simulink model "SVFB"  (R2024a)
settings: Solver=ode45  StartTime=0.0  StopTime=Tf  RelTol=1e-3
values from neighbouring files (symbols this model uses):
  A = [0 1; 880.87 0]    [main.m]
  B = [0; -9.9453]    [main.m]
  C = [708.27 0]    [main.m]
  K0 = place(A, B, p_desired_tracking)    [main.m]
  L_luemb = place(A', C', desired_poles)'    [main.m]
  S0_x0 = [10 0]'    [main.m]
undefined symbols (not defined in the file or in its folder): err
settings Model: Creator=aless  LastModifiedBy=Stefano

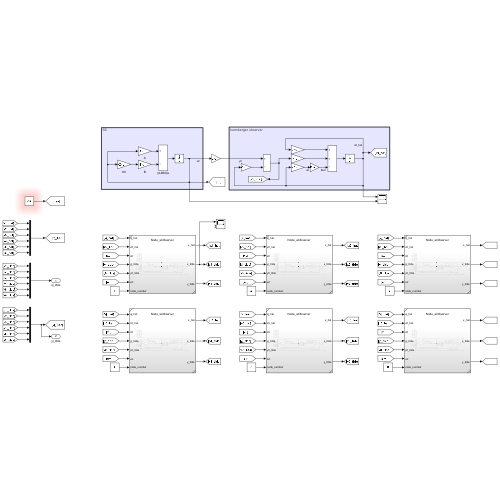
[thumbnail: Simulink's stored preview of the top-level diagram]
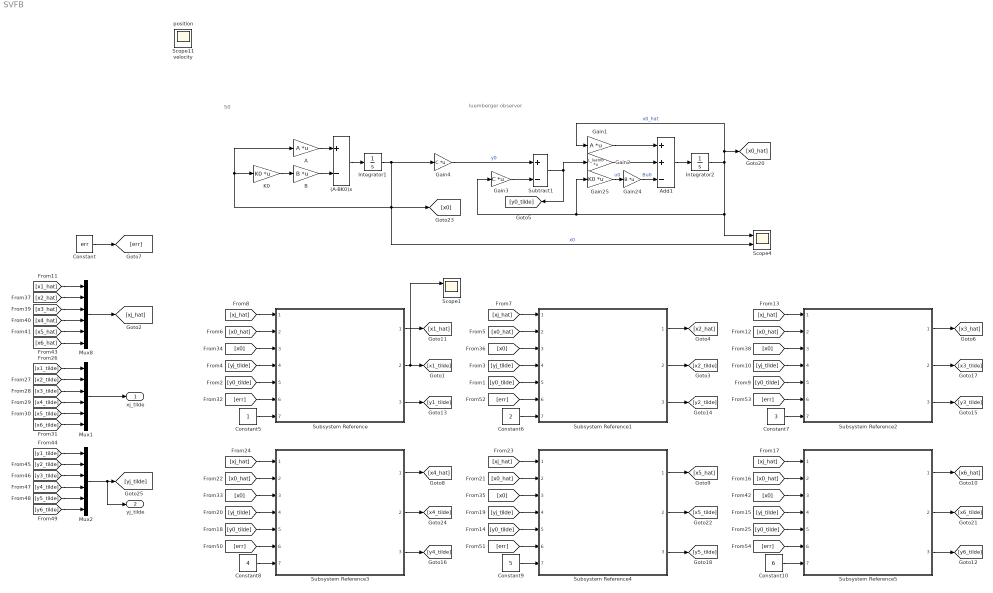
== system SVFB ==
  note: luemberger observer
  note: S0
  (A-BK0)x : Sum  Inputs=+-
  A : Gain  Gain=A  Multiplication=Matrix(K*u)
  Add1 : Sum  Inputs=++-
  B : Gain  Gain=B  Multiplication=Matrix(K*u)
  Constant : Constant  Value=err
  Constant10 : Constant  Value=6
  Constant5 : Constant
  Constant6 : Constant  Value=2
  Constant7 : Constant  Value=3
  Constant8 : Constant  Value=4
  Constant9 : Constant  Value=5
  Gain1 : Gain  Gain=A  Multiplication=Matrix(K*u)
  Gain2 : Gain  Gain=L_luemb  Multiplication=Matrix(K*u)
  Gain24 : Gain  Gain=B  Multiplication=Matrix(K*u)
  Gain25 : Gain  Gain=K0  Multiplication=Matrix(K*u)
  Gain3 : Gain  Gain=C  Multiplication=Matrix(K*u)
  Gain4 : Gain  Gain=C  Multiplication=Matrix(K*u)
  Integrator1 : Integrator  InitialCondition=S0_x0
  Integrator2 : Integrator  InitialCondition=S0_x0
  K0 : Gain  Gain=K0  Multiplication=Matrix(K*u)
  Mux1 : Mux  Inputs=6
  Mux2 : Mux  Inputs=6
  Mux8 : Mux  Inputs=6
  Scope1 : Scope  NumInputPorts=2
  Scope4 : Scope  NumInputPorts=2
  Subsystem Reference{,1..5} (6 alike) : Subsystem  ReferencedSubsystem=Node_wObserver
  Subtract1 : Sum  Inputs=+-
  xj_tilde : Outport
  yj_tilde : Outport  Port=2
  Scope11 : Scope
  position : Scope
  velocity : Scope
  wires:
  [x5_hat] -> Mux8/5
  [x3_hat] -> Mux8/3
  [x2_hat] -> Mux8/2
  [x6_hat] -> Mux8/6
  Mux8/1 -> [xj_hat]
  [x1_hat] -> Mux8/1
  [x4_hat] -> Mux8/4
  Mux1/1 -> xj_tilde/1
  [y0_tilde] -> Subsystem Reference/5
  [yj_tilde] -> Subsystem Reference/4
  [x0_hat] -> Subsystem Reference/2
  [xj_hat] -> Subsystem Reference/1
  Subsystem Reference/1 -> [x1_hat]
  [x0_hat] -> Subsystem Reference1/2
  Subsystem Reference1/1 -> [x2_hat]
  [xj_hat] -> Subsystem Reference1/1
  [y0_tilde] -> Subsystem Reference1/5
  [yj_tilde] -> Subsystem Reference1/4
  [x0_hat] -> Subsystem Reference2/2
  Subsystem Reference2/1 -> [x3_hat]
  [xj_hat] -> Subsystem Reference2/1
  [y0_tilde] -> Subsystem Reference2/5
  [yj_tilde] -> Subsystem Reference2/4
  [yj_tilde] -> Subsystem Reference5/4
  Subsystem Reference5/1 -> [x6_hat]
  [y0_tilde] -> Subsystem Reference5/5
  [xj_hat] -> Subsystem Reference5/1
  [x0_hat] -> Subsystem Reference5/2
  [x0_hat] -> Subsystem Reference3/2
  Subsystem Reference3/1 -> [x4_hat]
  [xj_hat] -> Subsystem Reference4/1
  Subsystem Reference4/1 -> [x5_hat]
  [yj_tilde] -> Subsystem Reference4/4
  [x0_hat] -> Subsystem Reference4/2
  [xj_hat] -> Subsystem Reference3/1
  [y0_tilde] -> Subsystem Reference3/5
  [y0_tilde] -> Subsystem Reference4/5
  [yj_tilde] -> Subsystem Reference3/4
  Subsystem Reference3/3 -> [y4_tilde]
  Subsystem Reference/3 -> [y1_tilde]
  Subsystem Reference1/3 -> [y2_tilde]
  Subsystem Reference4/3 -> [y5_tilde]
  Subsystem Reference5/3 -> [y6_tilde]
  Subsystem Reference2/3 -> [y3_tilde]
  [x6_tilde] -> Mux1/6
  [x5_tilde] -> Mux1/5
  [x4_tilde] -> Mux1/4
  [x3_tilde] -> Mux1/3
  [x2_tilde] -> Mux1/2
  [x1_tilde] -> Mux1/1
  Gain2/1 -> Add1/2
  Gain3/1 -> Subtract1/2
  Gain1/1 -> Add1/1
  Integrator1/1 -> Scope4/2, [x0], A/1, K0/1, Gain4/1  "x0"
  Add1/1 -> Integrator2/1
  B/1 -> (A-BK0)x/2
  (A-BK0)x/1 -> Integrator1/1
  A/1 -> (A-BK0)x/1
  Subtract1/1 -> [y0_tilde], Gain2/1
  K0/1 -> B/1
  Integrator2/1 -> [x0_hat], Gain1/1, Gain3/1, Gain25/1, Scope4/1  "x0_hat"
  Gain4/1 -> Subtract1/1  "y0"
  Subsystem Reference/2 -> Scope1/1, [x1_tilde]
  Subsystem Reference1/2 -> [x2_tilde]
  Subsystem Reference5/2 -> [x6_tilde]
  Subsystem Reference2/2 -> [x3_tilde]
  Subsystem Reference4/2 -> [x5_tilde]
  Subsystem Reference3/2 -> [x4_tilde]
  [x0] -> Subsystem Reference3/3
  [x0] -> Subsystem Reference/3
  [x0] -> Subsystem Reference4/3
  [x0] -> Subsystem Reference1/3
  [x0] -> Subsystem Reference2/3
  [x0] -> Subsystem Reference5/3
  [y4_tilde] -> Mux2/4
  [y5_tilde] -> Mux2/5
  [y1_tilde] -> Mux2/1
  [y2_tilde] -> Mux2/2
  [y3_tilde] -> Mux2/3
  Mux2/1 -> yj_tilde/1, [yj_tilde]
  [y6_tilde] -> Mux2/6
  Gain25/1 -> Gain24/1  "u0"
  Gain24/1 -> Add1/3  "Bu0"
  Constant/1 -> [err]
  Constant5/1 -> Subsystem Reference/7
  [err] -> Subsystem Reference/6
  Constant8/1 -> Subsystem Reference3/7
  [err] -> Subsystem Reference3/6
  Constant9/1 -> Subsystem Reference4/7
  [err] -> Subsystem Reference4/6
  Constant6/1 -> Subsystem Reference1/7
  Constant10/1 -> Subsystem Reference5/7
  Constant7/1 -> Subsystem Reference2/7
  [err] -> Subsystem Reference1/6
  [err] -> Subsystem Reference2/6
  [err] -> Subsystem Reference5/6
